simulink model "scheme"  (R2024a)
settings: Solver=VariableStepAuto  StartTime=0.0  StopTime=40  RelTol=1e-3
settings Model: Creator=ventus  LastModifiedBy=ventus

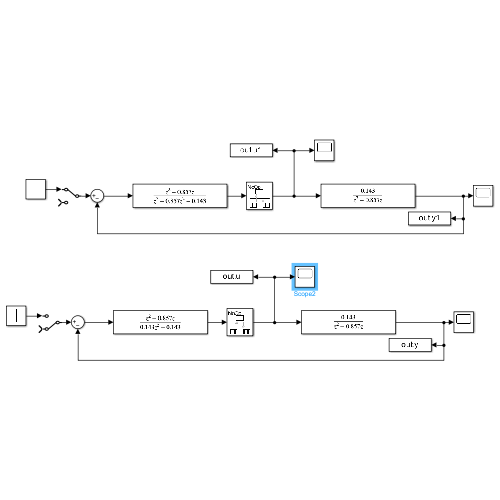
[thumbnail: Simulink's stored preview of the top-level diagram]
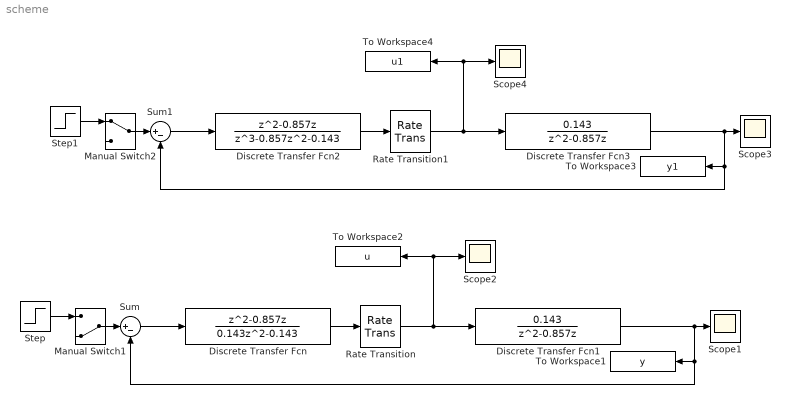
== system scheme ==
  Discrete Transfer Fcn : DiscreteTransferFcn  Numerator=[1 -0.857 0]  Denominator=[0.143 0 -0.143]
  Discrete Transfer Fcn1 : DiscreteTransferFcn  Numerator=[0.143]  Denominator=[1 -0.857 0]
  Discrete Transfer Fcn2 : DiscreteTransferFcn  Numerator=[1 -0.857 0]  Denominator=[1 -0.857 0 -0.143]
  Discrete Transfer Fcn3 : DiscreteTransferFcn  Numerator=[0.143]  Denominator=[1 -0.857 0]
  Manual Switch1 : ManualSwitch  CurrentSetting=0
  Manual Switch2 : ManualSwitch
  Rate Transition : RateTransition  OutPortSampleTime=1
  Rate Transition1 : RateTransition  OutPortSampleTime=1
  Scope{1..4} (4 alike) : Scope
  Step : Step  SampleTime=0
  Step1 : Step  SampleTime=0
  Sum : Sum  Inputs=|+-
  Sum1 : Sum  Inputs=|+-
  To Workspace1 : ToWorkspace  VariableName=y  SaveFormat=Timeseries  SampleTime=-1
  To Workspace2 : ToWorkspace  VariableName=u  SaveFormat=Timeseries  SampleTime=-1
  To Workspace3 : ToWorkspace  VariableName=y1  SaveFormat=Timeseries  SampleTime=-1
  To Workspace4 : ToWorkspace  VariableName=u1  SaveFormat=Timeseries  SampleTime=-1
  wires:
  Step/1 -> Manual Switch1/1
  Discrete Transfer Fcn1/1 -> Scope1/1, To Workspace1/1, Sum/2
  Sum/1 -> Discrete Transfer Fcn/1
  Manual Switch1/1 -> Sum/1
  Discrete Transfer Fcn/1 -> Rate Transition/1
  Rate Transition/1 -> To Workspace2/1, Scope2/1, Discrete Transfer Fcn1/1
  Discrete Transfer Fcn2/1 -> Rate Transition1/1
  Rate Transition1/1 -> To Workspace4/1, Scope4/1, Discrete Transfer Fcn3/1
  Manual Switch2/1 -> Sum1/1
  Step1/1 -> Manual Switch2/1
  Sum1/1 -> Discrete Transfer Fcn2/1
  Discrete Transfer Fcn3/1 -> Scope3/1, To Workspace3/1, Sum1/2
